simulink model "simple_arda_mpc"  (R2021b)
settings: Solver=FixedStepAuto  StartTime=0  StopTime=10000  FixedStep=0.1  RelTol=1e-3
PreLoadFcn:
  | % Setup model parameters
  |                 % Sample time
  |                 %Ts = 0.1;
  |                 % Simulation stop time ("TimeOut")
  |                 %stop_time = 8000;
  |                 % Temperature
  |                 %T_init = 20 + 273.1755;
  |                % T_final = 294.1755;
  |               %  T_env = 20 + 273.15; %#ok<*NASGU>
  |              %   % Heater
  |                 %u_volts_heater_init = 0; % volts
  |                 % Pressure
  |                 %p_init = 101.325; % kPa
  |                 %p_env = 101.325; % kPa
  |                 % Relative humidity and steam
  |                 %phi_init = 0.4987;
  |                 %phi_final = 0.6;
  |                 %phi_env = 0.1;
  |                 %u_steam_init = 0;
  |                 %T_steam = 130 + 273.15;
  |                 % Volumetric flow rate
  |                 %u_volts_fan_init = 1;
  |                 %flow_init = 5.8e-3;
  |                 %flow_final = 0.18;
  |                 % Smooth ramp input parameters
  |                 %smooth_step_heater = make_smooth_step(0, T_init, T_final, Ts, stop_time, 'T_g');
  |                 %smooth_step_steam = make_smooth_step(0, phi_init, phi_final, Ts, stop_time, 'phi');
  |                 %smooth_step_fan = make_smooth_step(0, flow_init, flow_final, Ts, stop_time, 'flow');
  |                 % Parameters to vary for linearization
  |                 % Pipes
  |                 %pipe_length1 = 1; % meters
  |                 %pipe_length2 = 1;
  |                 %pipe_length3 = 1;
  |                 %pipe_cross_sectional_area1 = pi*(2*2.54/2)^2; % cm^2
  |                 %pipe_cross_sectional_area2 = pi*(2*2.54/2)^2;
  |                 %pipe_cross_sectional_area3 = pi*(2*2.54/2)^2;
  |                 %pipe_hydraulic_diameter1 = 2*2.54; %cm
  |                 %pipe_hydraulic_diameter2 = 2*2.54; %cm
  |                 %pipe_hydraulic_diameter3 = 2*2.54; %cm
  |                 % Thermal masses
  |                 %thermal_mass1 = 1; % kg
  |                 %thermal_mass2 = 1; % kg
  |                 %thermal_mass3 = 1; % kg
  |                 %thermal_mass4 = 1; % kg
  |                 %thermal_mass5 = 1; % kg
  |                 %specific_heat1 = 447; % J/(K*kg)
  |                 %specific_heat2 = 447; % J/(K*kg)
  |                 %specific_heat3 = 447; % J/(K*kg)
  |                 %specific_heat4 = 447; % J/(K*kg)
  |                 %specific_heat5 = 447; % J/(K*kg)
InitFcn:
  | load('bob.mat')
libraries: simulink x3, mpclib x1
settings Model: DataDictionary=data_dictionary1.sldd  Creator=dmeissner  LastModifiedBy=dmeissner
settings SolverCC: ZeroCrossAlgorithm=Adaptive
settings DataIOCC: DSMLogging=off
settings DebuggingCC: ModelReferenceIOMsg=warning  ModelReferenceVersionMismatchMessage=warning  ModelReferenceIOMismatchMessage=warning  ModelReferenceNoExplicitFinalValueMsg=warning

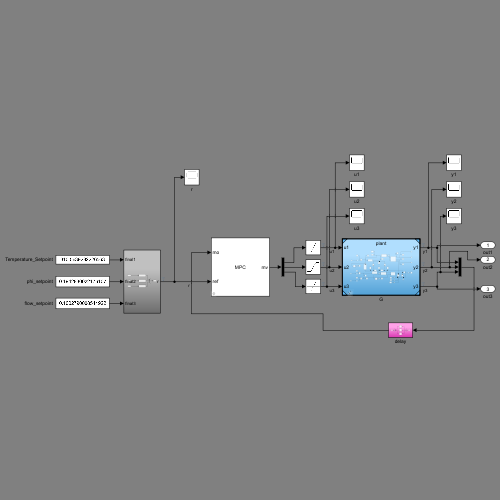
[thumbnail: Simulink's stored preview of the top-level diagram]
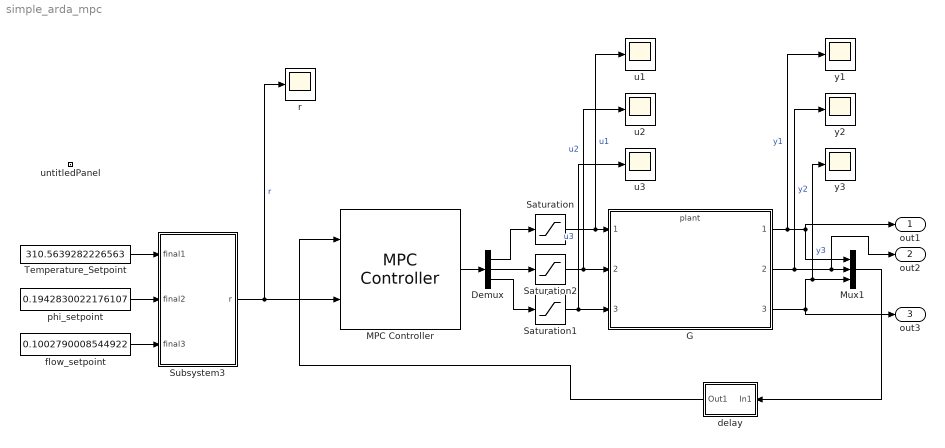
== system simple_arda_mpc ==
  Demux : Demux  Outputs=3
  G : ModelReference  ModelNameDialog=plant.slx  SimulationMode=Normal  ModelReferenceVersion=1.120
  MPC Controller : mpclib/MPC Controller  SCDEnableBlockLinearizationSpecification=on  mpcobj=bob.controller.mpc1  x0=bob.controller.mpc1_initial_state  is_multiple=0  enable_value=0  return_u0=off  updateMPCinCallerWorkspace=on  md_inport=off  mv_inport=off  uref_inport=off  return_cost=off  return_mvseq=off  return_qpstatus=off  return_xseq=off  return_state=off  return_ovseq=off  state_inport=off  umin_inport=off  umax_inport=off  ymin_inport=off  ymax_inport=off  cc_inport=off  ywt_inport=off  uwt_inport=off  duwt_inport=off  rhoeps_inport=off  pm_inport=off  MaximumP=10  HorizonChoice=FixedHorizon  n_ts=1  n_p=10  n_mv=3  n_md=0  n_ud=0  n_mo=3  n_uo=0  BlockDataType=double  SampleTimeInherited=off  switch_inport=off
  Mux1 : Mux  Inputs=3
  Saturation : Saturate  UpperLimit=460  LowerLimit=0
  Saturation1 : Saturate  UpperLimit=460  LowerLimit=0
  Saturation2 : Saturate  UpperLimit=0.06  LowerLimit=0
  Subsystem3 : Subsystem
  Temperature_Setpoint : Constant  Value=310.5639282226563
  delay : Subsystem
  flow_setpoint : Constant  Value=0.1002790008544922
  phi_setpoint : Constant  Value=0.1942830022176107
  r : Scope
  u1 : Scope
  u2 : Scope
  u3 : Scope
  untitledPanel : Subsystem  Tag=HiddenForWebPanel  IsWebBlockPanel=on
  y1 : Scope
  y2 : Scope
  y3 : Scope
  out1 : Outport
  out2 : Outport  Port=2
  out3 : Outport  Port=3
  wires:
  G/2 -> y2/1, out2/1, Mux1/2  "y2"
  G/1 -> y1/1, Mux1/1, out1/1  "y1"
  G/3 -> y3/1, Mux1/3, out3/1  "y3"
  Saturation/1 -> u1/1, G/1  "u1"
  Saturation2/1 -> u2/1, G/2  "u2"
  Saturation1/1 -> u3/1, G/3  "u3"
  Mux1/1 -> delay/1(In1)
  delay/1(Out1) -> MPC Controller/1
  Subsystem3/1(r) -> r/1, MPC Controller/2  "r"
  Demux/1 -> Saturation/1
  Demux/2 -> Saturation2/1
  Demux/3 -> Saturation1/1
  MPC Controller/1 -> Demux/1
  Temperature_Setpoint/1 -> Subsystem3/1(final1)
  phi_setpoint/1 -> Subsystem3/2(final2)
  flow_setpoint/1 -> Subsystem3/3(final3)

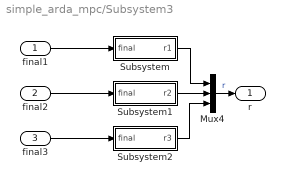
== system simple_arda_mpc/Subsystem3 ==
  final1 : Inport
  final2 : Inport  Port=2
  final3 : Inport  Port=3
  Mux4 : Mux  Inputs=3
  Subsystem : Subsystem
  Subsystem1 : Subsystem
  Subsystem2 : Subsystem
  r : Outport
  wires:
  final2/1 -> Subsystem1/1(final)
  Subsystem1/1(r2) -> Mux4/2
  Subsystem2/1(r3) -> Mux4/3
  Subsystem/1(r1) -> Mux4/1
  final1/1 -> Subsystem/1(final)
  final3/1 -> Subsystem2/1(final)
  Mux4/1 -> r/1  "r"

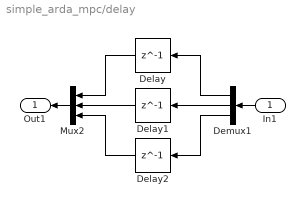
== system simple_arda_mpc/delay ==
  In1 : Inport
  Delay : Delay  DelayLength=1
  Delay1 : Delay  DelayLength=1
  Delay2 : Delay  DelayLength=1
  Demux1 : Demux  Outputs=3
  Mux2 : Mux  Inputs=3
  Out1 : Outport
  wires:
  Mux2/1 -> Out1/1
  Demux1/2 -> Delay1/1
  In1/1 -> Demux1/1
  Delay1/1 -> Mux2/2
  Demux1/3 -> Delay2/1
  Delay/1 -> Mux2/1
  Demux1/1 -> Delay/1
  Delay2/1 -> Mux2/3

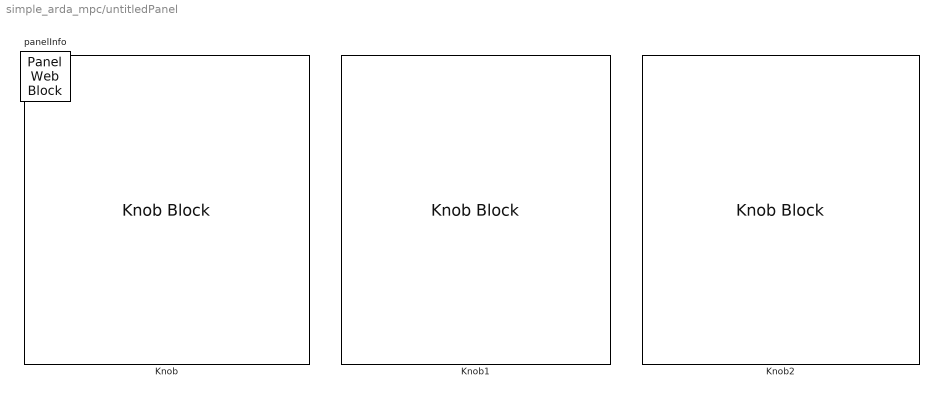
== system simple_arda_mpc/untitledPanel ==
  Knob : KnobBlock  Tag=HiddenForWebPanel  PanelInfo="{\"panelId\":\"panelId-06cae6c1-80a6-464e-a568-f56bf80fba14\",\"type\":\"panelChild\",\"version\":\"2019b\",\"zIndex\":1500004}"  ScaleMin=290  ScaleMax=450  TickInterval=10
  Knob1 : KnobBlock  Tag=HiddenForWebPanel  PanelInfo="{\"panelId\":\"panelId-06cae6c1-80a6-464e-a568-f56bf80fba14\",\"type\":\"panelChild\",\"version\":\"2019b\",\"zIndex\":1500002}"  ScaleMax=1  TickInterval=0.1
  Knob2 : KnobBlock  Tag=HiddenForWebPanel  PanelInfo="{\"panelId\":\"panelId-06cae6c1-80a6-464e-a568-f56bf80fba14\",\"type\":\"panelChild\",\"version\":\"2019b\",\"zIndex\":1500006}"  ScaleMax=0.18  TickInterval=0.01
  panelInfo : PanelWebBlock  Tag=HiddenForWebPanel  PanelInfo="{\"compacted\":false,\"height\":349,\"isActiveTab\":true,\"left\":49,\"name\":\"Panel\",\"panelId\":\"panelId-06cae6c1-80a6-464e-a568-f56bf80fba14\",\"tabIndex\":0,\"tabbedSetId\":\"tabbedSet4008599384\",\"top\":23,\"type\":\"panel\",\"version\":\"2019b\",\"visible\":true,\"width\":935,\"zIndex\":1500002}"  PanelSnapshot=<binary blob, 164980 chars, not shown>

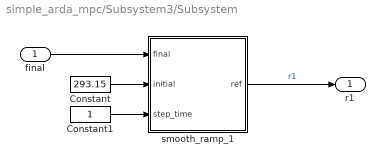
== system simple_arda_mpc/Subsystem3/Subsystem ==
  final : Inport
  Constant : Constant  Value=293.15
  Constant1 : Constant
  smooth_ramp_1 : Subsystem
  r1 : Outport
  wires:
  Constant1/1 -> smooth_ramp_1/3(step_time)
  smooth_ramp_1/1(ref) -> r1/1  "r1"
  Constant/1 -> smooth_ramp_1/2(initial)
  final/1 -> smooth_ramp_1/1(final)

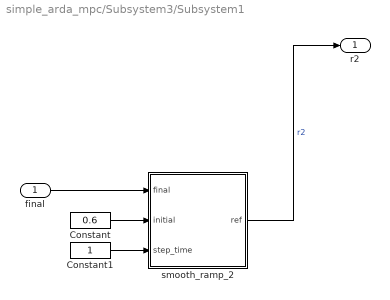
== system simple_arda_mpc/Subsystem3/Subsystem1 ==
  final : Inport
  Constant : Constant  Value=0.6
  Constant1 : Constant
  smooth_ramp_2 : Subsystem
  r2 : Outport
  wires:
  final/1 -> smooth_ramp_2/1(final)
  Constant/1 -> smooth_ramp_2/2(initial)
  smooth_ramp_2/1(ref) -> r2/1  "r2"
  Constant1/1 -> smooth_ramp_2/3(step_time)

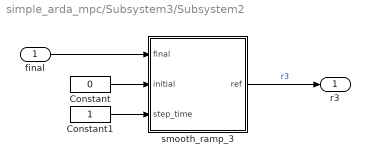
== system simple_arda_mpc/Subsystem3/Subsystem2 ==
  final : Inport
  Constant : Constant  Value=0
  Constant1 : Constant
  smooth_ramp_3 : Subsystem
  r3 : Outport
  wires:
  Constant1/1 -> smooth_ramp_3/3(step_time)
  smooth_ramp_3/1(ref) -> r3/1  "r3"
  Constant/1 -> smooth_ramp_3/2(initial)
  final/1 -> smooth_ramp_3/1(final)

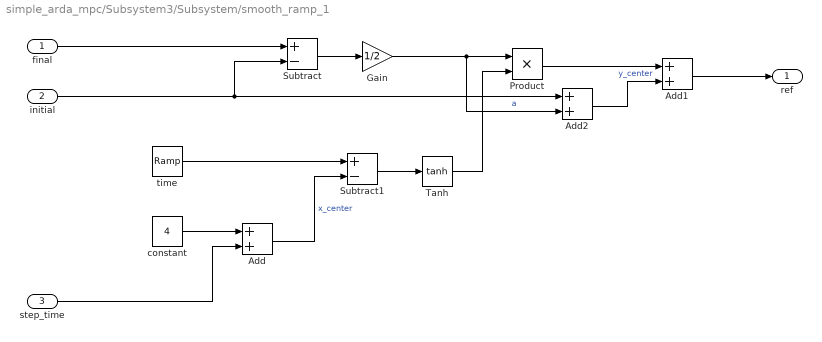
== system simple_arda_mpc/Subsystem3/Subsystem/smooth_ramp_1 ==
  final : Inport
  initial : Inport  Port=2
  step_time : Inport  Port=3
  Add : Sum
  Add1 : Sum
  Add2 : Sum
  Gain : Gain  Gain=1/2
  Product : Product
  Subtract : Sum  Inputs=+-
  Subtract1 : Sum  Inputs=+-
  Tanh : Trigonometry  Operator=tanh
  constant : Constant  Value=4
  time : simulink/Sources/Ramp  slope=1  start=0  InitialOutput=0
  ref : Outport
  wires:
  final/1 -> Subtract/1
  initial/1 -> Add2/1, Subtract/2
  Subtract/1 -> Gain/1
  Gain/1 -> Add2/2, Product/1  "a"
  constant/1 -> Add/1
  step_time/1 -> Add/2
  Add/1 -> Subtract1/2  "x_center"
  time/1 -> Subtract1/1
  Subtract1/1 -> Tanh/1
  Tanh/1 -> Product/2
  Product/1 -> Add1/1
  Add2/1 -> Add1/2  "y_center"
  Add1/1 -> ref/1

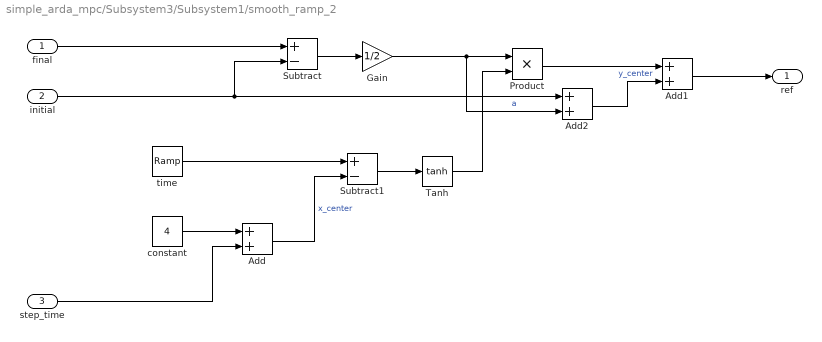
== system simple_arda_mpc/Subsystem3/Subsystem1/smooth_ramp_2 ==
  final : Inport
  initial : Inport  Port=2
  step_time : Inport  Port=3
  Add : Sum
  Add1 : Sum
  Add2 : Sum
  Gain : Gain  Gain=1/2
  Product : Product
  Subtract : Sum  Inputs=+-
  Subtract1 : Sum  Inputs=+-
  Tanh : Trigonometry  Operator=tanh
  constant : Constant  Value=4
  time : simulink/Sources/Ramp  slope=1  start=0  InitialOutput=0
  ref : Outport
  wires:
  Add1/1 -> ref/1
  Add2/1 -> Add1/2  "y_center"
  Product/1 -> Add1/1
  Tanh/1 -> Product/2
  Subtract1/1 -> Tanh/1
  time/1 -> Subtract1/1
  Add/1 -> Subtract1/2  "x_center"
  step_time/1 -> Add/2
  constant/1 -> Add/1
  Gain/1 -> Product/1, Add2/2  "a"
  Subtract/1 -> Gain/1
  initial/1 -> Subtract/2, Add2/1
  final/1 -> Subtract/1

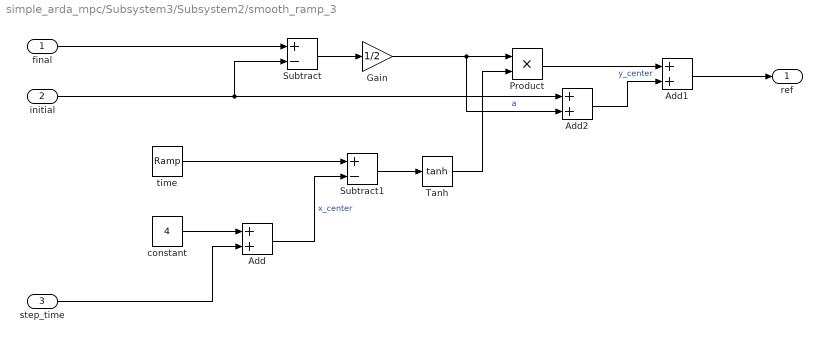
== system simple_arda_mpc/Subsystem3/Subsystem2/smooth_ramp_3 ==
  final : Inport
  initial : Inport  Port=2
  step_time : Inport  Port=3
  Add : Sum
  Add1 : Sum
  Add2 : Sum
  Gain : Gain  Gain=1/2
  Product : Product
  Subtract : Sum  Inputs=+-
  Subtract1 : Sum  Inputs=+-
  Tanh : Trigonometry  Operator=tanh
  constant : Constant  Value=4
  time : simulink/Sources/Ramp  slope=1  start=0  InitialOutput=0
  ref : Outport
  wires:
  final/1 -> Subtract/1
  initial/1 -> Add2/1, Subtract/2
  Subtract/1 -> Gain/1
  Gain/1 -> Add2/2, Product/1  "a"
  constant/1 -> Add/1
  step_time/1 -> Add/2
  Add/1 -> Subtract1/2  "x_center"
  time/1 -> Subtract1/1
  Subtract1/1 -> Tanh/1
  Tanh/1 -> Product/2
  Product/1 -> Add1/1
  Add2/1 -> Add1/2  "y_center"
  Add1/1 -> ref/1
